simulink model "arduino_test"  (R2018b)
settings: Solver=FixedStepAuto  StartTime=0.0  StopTime=200  RelTol=1e-3  EnableMultiTasking=on
libraries: arduinolib x3, simulink x1
settings Model: EnablePacing=on  ExtModeTrigDuration=2  Creator=benkl  LastModifiedBy=benkl
settings SolverCC: AutoInsertRateTranBlk=on
settings OptimizationCC: EnhancedBackFolding=on  PassReuseOutputArgsAs=Individual arguments  MaxStackSize=64  OptimizeBlockOrder=speed  DifferentSizesBufferReuse=on  OptimizationCustomize=off
settings DebuggingCC: ParameterTunabilityLossMsg=error
settings HardwareCC: ProdBitPerInt=16  ProdBitPerPointer=16  ProdBitPerSizeT=16  ProdBitPerPtrDiffT=16  ProdLargestAtomicFloat=None  ProdWordSize=8  ProdHWDeviceType=Atmel->AVR
settings SFSimCC: MATLABDynamicMemAlloc=off
settings RTWCC: SystemTargetFile=ert.tlc  HardwareBoard=Arduino Uno  TemplateMakefile=ert_default_tmf  GenerateReport=on  Toolchain=Arduino AVR  BuildConfiguration=Faster Runs  IncludeHyperlinkInReport=on  LaunchReport=on  GenerateTraceInfo=on  GenerateTraceReport=on  GenerateTraceReportSl=on  GenerateTraceReportSf=on  GenerateTraceReportEml=on
settings CodeAppCC: ForceParamTrailComments=on  IgnoreCustomStorageClasses=off  OperatorAnnotations=on  SimulinkDataObjDesc=on  SFDataObjDesc=on  InsertBlockDesc=on
settings ERTTargetCC: SupportContinuousTime=on  SupportVariableSizeSignals=on

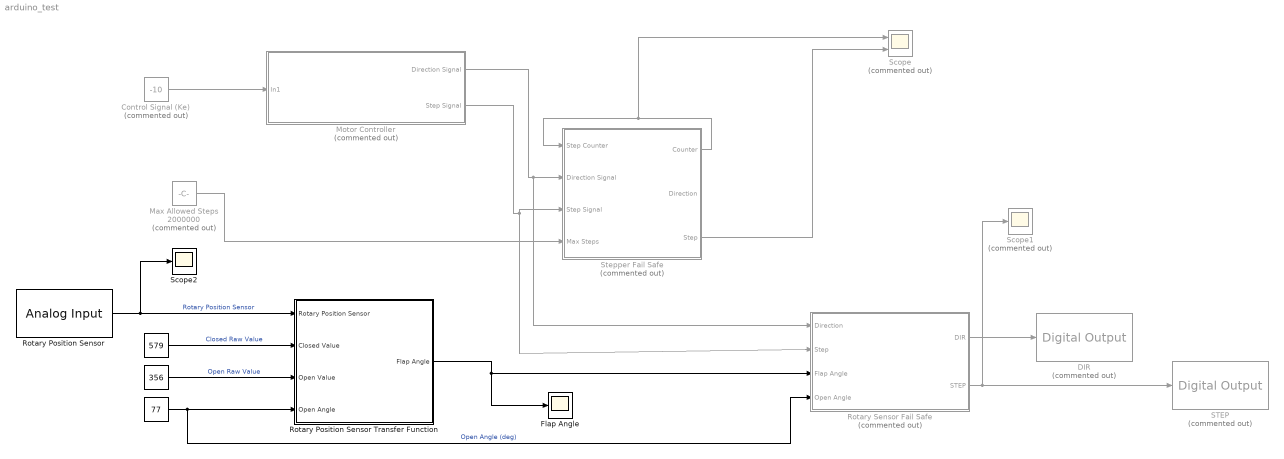
== system arduino_test ==
  " " : Constant  Value=579
  "  " : Constant  Value=77
  " " : Constant  Value=356
  Control Signal (Ke) : Constant  Commented=on  Value=-10
  DIR : arduinolib/Digital Output  Commented=on  pinNumber=2  blockPlatform=arduino
  Flap Angle : Scope
  Max Allowed Steps : Constant  Commented=on  Value=2000000
  Motor Controller : Subsystem  Commented=on
  Rotary Position Sensor : arduinolib/Analog Input  pinNumber=4  ReadResultsOnly=off  ConversionTriggerSource=Software  ExternalTriggerType=uint32(0)  OutputDataType=uint16  EnableConversionCompleteNotify=off  EnableOuputStatus=off  SampleTime=0.01  blockPlatform=arduino
  Rotary Position Sensor Transfer Function : Subsystem
  Rotary Sensor Fail Safe : Subsystem  Commented=on
  STEP : arduinolib/Digital Output  Commented=on  pinNumber=13  blockPlatform=arduino
  Scope : Scope  Commented=on  NumInputPorts=2
  Scope1 : Scope  Commented=on
  Scope2 : Scope
  Stepper Fail Safe : Subsystem  Commented=on
  wires:
  " "/1 -> Rotary Position Sensor Transfer Function/2(Closed Value)  "Closed Raw Value"
  " "/1 -> Rotary Position Sensor Transfer Function/3(Open Value)  "Open Raw Value"
  Motor Controller/2(Step Signal) -> Rotary Sensor Fail Safe/2(Step), Stepper Fail Safe/3(Step Signal)
  Motor Controller/1(Direction Signal) -> Rotary Sensor Fail Safe/1(Direction), Stepper Fail Safe/2(Direction Signal)
  Control Signal (Ke)/1 -> Motor Controller/1(In1)
  Rotary Position Sensor Transfer Function/1(Flap Angle) -> Flap Angle/1, Rotary Sensor Fail Safe/3(Flap Angle)
  Rotary Position Sensor/1 -> Scope2/1, Rotary Position Sensor Transfer Function/1(Rotary Position Sensor)  "Rotary Position Sensor"
  Stepper Fail Safe/1(Counter) -> Scope/1, Stepper Fail Safe/1(Step Counter)
  Stepper Fail Safe/3(Step) -> Scope/2
  Max Allowed Steps/1 -> Stepper Fail Safe/4(Max Steps)
  "  "/1 -> Rotary Sensor Fail Safe/4(Open Angle), Rotary Position Sensor Transfer Function/4(Open Angle)  "Open Angle (deg)"
  Rotary Sensor Fail Safe/2(STEP) -> Scope1/1, STEP/1
  Rotary Sensor Fail Safe/1(DIR) -> DIR/1

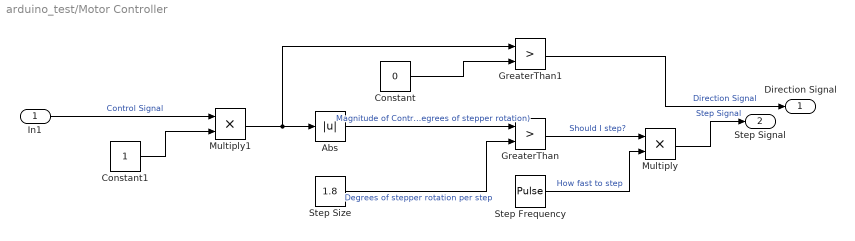
== system arduino_test/Motor Controller ==
  In1 : Inport
  Abs : Abs
  Constant : Constant  Value=0
  Constant1 : Constant
  GreaterThan : RelationalOperator  Operator=>  OutDataTypeStr=boolean  RndMeth=Simplest
  GreaterThan1 : RelationalOperator  Operator=>  OutDataTypeStr=boolean  RndMeth=Simplest
  Multiply : Product
  Multiply1 : Product
  Step Frequency : DiscretePulseGenerator  PulseType=Time based  Period=1  PulseWidth=50
  Step Size : Constant  Value=1.8
  Direction Signal : Outport
  Step Signal : Outport  Port=2
  wires:
  Abs/1 -> GreaterThan/1  "Magnitude of Control Signal (degrees of stepper rotation)"
  Constant/1 -> GreaterThan1/2
  Step Size/1 -> GreaterThan/2  "Degrees of stepper rotation per step"
  In1/1 -> Multiply1/1  "Control Signal"
  Step Frequency/1 -> Multiply/2  "How fast to step"
  GreaterThan/1 -> Multiply/1  "Should I step?"
  Multiply/1 -> Step Signal/1  "Step Signal"
  GreaterThan1/1 -> Direction Signal/1  "Direction Signal"
  Multiply1/1 -> GreaterThan1/1, Abs/1
  Constant1/1 -> Multiply1/2

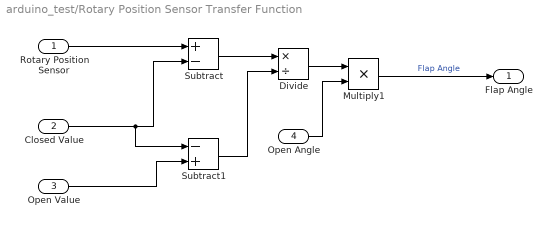
== system arduino_test/Rotary Position Sensor Transfer Function ==
  Rotary Position Sensor : Inport
  Closed Value : Inport  Port=2
  Open Value : Inport  Port=3
  Open Angle : Inport  Port=4
  Divide : Product  Inputs=*/
  Multiply1 : Product
  Subtract : Sum  Inputs=+-
  Subtract1 : Sum  Inputs=-+
  Flap Angle : Outport
  wires:
  Subtract/1 -> Divide/1
  Closed Value/1 -> Subtract1/1, Subtract/2
  Divide/1 -> Multiply1/1
  Open Angle/1 -> Multiply1/2
  Subtract1/1 -> Divide/2
  Rotary Position Sensor/1 -> Subtract/1
  Open Value/1 -> Subtract1/2
  Multiply1/1 -> Flap Angle/1  "Flap Angle"

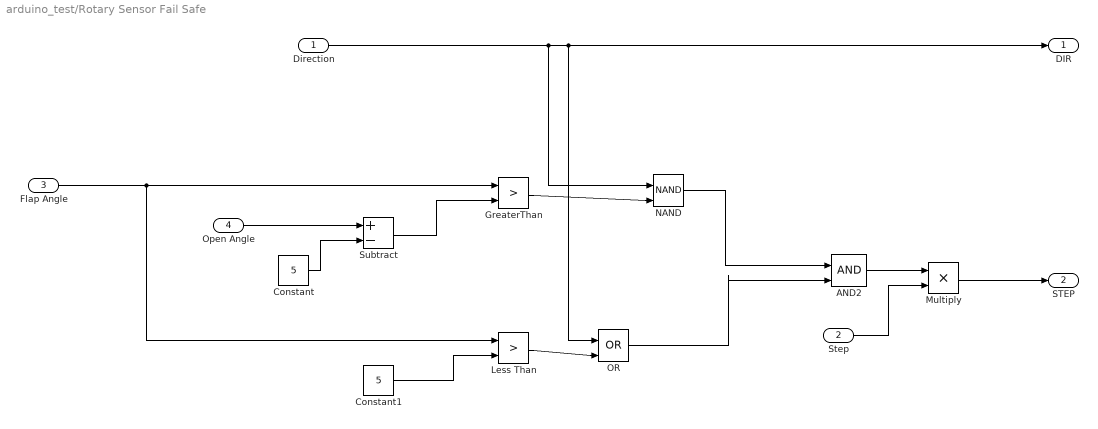
== system arduino_test/Rotary Sensor Fail Safe ==
  Direction : Inport
  Step : Inport  Port=2
  Flap Angle : Inport  Port=3
  Open Angle : Inport  Port=4
  AND2 : Logic  IconShape=distinctive  AllPortsSameDT=off  OutDataTypeStr=boolean
  Constant : Constant  Value=5
  Constant1 : Constant  Value=5
  GreaterThan : RelationalOperator  Operator=>  OutDataTypeStr=boolean  RndMeth=Simplest
  Less Than : RelationalOperator  Operator=>  OutDataTypeStr=boolean  RndMeth=Simplest
  Multiply : Product
  NAND : Logic  Operator=NAND  IconShape=distinctive  AllPortsSameDT=off  OutDataTypeStr=boolean
  OR : Logic  Operator=OR  IconShape=distinctive  AllPortsSameDT=off  OutDataTypeStr=boolean
  Subtract : Sum  Inputs=+-
  DIR : Outport
  STEP : Outport  Port=2
  wires:
  Flap Angle/1 -> Less Than/1, GreaterThan/1
  Constant/1 -> Subtract/2
  Open Angle/1 -> Subtract/1
  Subtract/1 -> GreaterThan/2
  GreaterThan/1 -> NAND/2
  Multiply/1 -> STEP/1
  Step/1 -> Multiply/2
  Direction/1 -> NAND/1, OR/1, DIR/1
  AND2/1 -> Multiply/1
  Less Than/1 -> OR/2
  Constant1/1 -> Less Than/2
  OR/1 -> AND2/2
  NAND/1 -> AND2/1

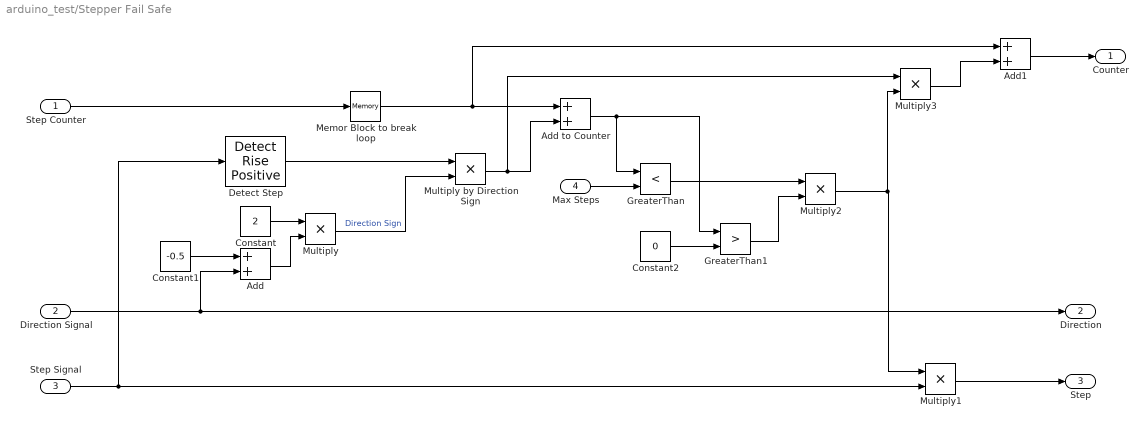
== system arduino_test/Stepper Fail Safe ==
  Step Counter : Inport
  Direction Signal : Inport  Port=2
  Step Signal : Inport  Port=3
  Max Steps : Inport  Port=4
  Add : Sum
  Add to Counter : Sum
  Add1 : Sum
  Constant : Constant  Value=2
  Constant1 : Constant  Value=-0.5
  Constant2 : Constant  Value=0
  Detect Step : simulink/Logic and Bit Operations/Detect Rise Positive  vinit=0  OutDataTypeStr=uint8
  GreaterThan : RelationalOperator  Operator=<  OutDataTypeStr=boolean  RndMeth=Simplest
  GreaterThan1 : RelationalOperator  Operator=>  OutDataTypeStr=boolean  RndMeth=Simplest
  Memor Block to break loop : Memory
  Multiply{,1..3} (4 alike) : Product
  Multiply by Direction Sign : Product
  Counter : Outport
  Direction : Outport  Port=2
  Step : Outport  Port=3
  wires:
  Direction Signal/1 -> Add/2, Direction/1
  Add to Counter/1 -> GreaterThan1/1, GreaterThan/1
  Detect Step/1 -> Multiply by Direction Sign/1
  Multiply by Direction Sign/1 -> Multiply3/1, Add to Counter/2
  Step Counter/1 -> Memor Block to break loop/1
  Memor Block to break loop/1 -> Add1/1, Add to Counter/1
  Multiply/1 -> Multiply by Direction Sign/2  "Direction Sign"
  Add/1 -> Multiply/2
  Constant1/1 -> Add/1
  Constant/1 -> Multiply/1
  Max Steps/1 -> GreaterThan/2
  Multiply1/1 -> Step/1
  GreaterThan/1 -> Multiply2/1
  Multiply2/1 -> Multiply3/2, Multiply1/1
  GreaterThan1/1 -> Multiply2/2
  Constant2/1 -> GreaterThan1/2
  Step Signal/1 -> Detect Step/1, Multiply1/2
  Add1/1 -> Counter/1
  Multiply3/1 -> Add1/2
